simulink model "p2_sync_cosim"  (Simulink 6.4)
settings: Solver=FixedStepDiscrete  SolverMode=SingleTasking  StartTime=0.0  StopTime=0.4  RelTol=1e-3
undefined symbols (not defined in the file or in its folder): pipeline_prec
libraries: modelsimlib x1
settings Model: LastModifiedBy=Administrador

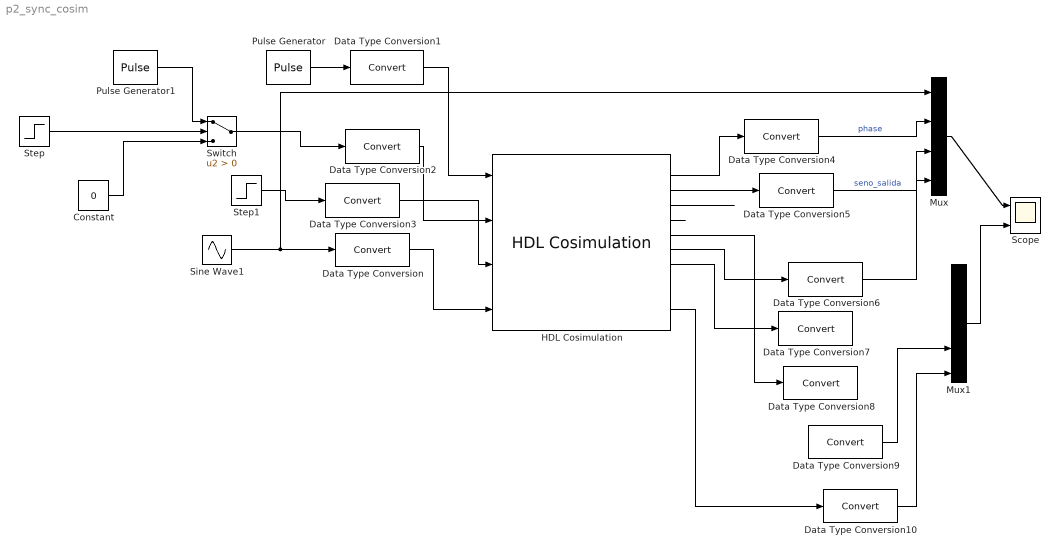
== system p2_sync_cosim ==
  Constant : Constant  Value=0  OutDataType=sfix(16)  ConRadixGroup=Use specified scaling  OutScaling=2^0  SampleTime=-1  FramePeriod=inf
  Data Type Conversion : DataTypeConversion  OutDataTypeMode=Specify via dialog  OutScaling=2^(-pipeline_prec)  RndMeth=Nearest  SaturateOnIntegerOverflow=on
  Data Type Conversion1 : DataTypeConversion  OutDataTypeMode=boolean
  Data Type Conversion{4..10} (7 alike) : DataTypeConversion
  Data Type Conversion2 : DataTypeConversion  OutDataTypeMode=boolean
  Data Type Conversion3 : DataTypeConversion  OutDataTypeMode=boolean
  HDL Cosimulation : modelsimlib/HDL Cosimulation  DialogController=modelsimddg.CoSim  DialogControllerArgs=DataTag0  PortPaths=/p2_sync/clk;/p2_sync/sample;/p2_sync/rst;/p2_sync/in_signal;/p2_sync/phase;/p2_sync/out_signal;/p2_sync/ampl;/p2_sync/done;/p2_sync/freq2phase_out_s;/p2_sync/phase_error_s;/p2_sync/in_cos_mul_out_s;/p2_sync/in_signal_reg_out_s;/p2_sync/sin_speedup_reg_out_s;/p2_sync/cos_speedup_reg_out_s  PortModes=[1 1 1 1 2 2 2 2 2 2 2 2 2 2 ]  PortTimes=[1,1,1,1,1e-5,1e-5,1e-5,1,1e-5,1e-5,1e-5,1e-5,1e-5,1e-5]  PortSigns=[-1 -1 -1 -1 1 1 1 -1 1 1 1 1 1 1 ]  PortFracLengths=[0,0,0,0,pipeline_prec,pipeline_prec,pipeline_prec,0,pipeline_prec,pipeline_prec,pipeline_prec,pipeline_prec,pipeline_prec,pipeline_prec]  CommLocal=on  CommSharedMemory=off  CommPortNumber=4449  CommShowInfo=on  ClockModes=[]  ClockTimes=[]  TclPreSimCommand="echo \"Running Simulink Cosimulation block.\""  TclPostSimCommand="echo \"done\""  TimingMode=s  TimingScaleFactor=1  idxCellArray={'UNUSED_VAR'}
  Mux : Mux
  Mux1 : Mux  Inputs=5
  Pulse Generator : DiscretePulseGenerator  PulseType=Time based  Period=1/(1e6)  PulseWidth=50
  Pulse Generator1 : DiscretePulseGenerator  PulseType=Time based  Period=0.1e-3  PulseWidth=2
  Scope : Scope  NumInputPorts=2
      settings: YMin=-3.5~-1  YMax=3.5~2  MaxDataPoints=500000
  Sine Wave1 : Sin  Frequency=2*pi*50  Phase=1
  Step : Step  Time=4*(1/1e6)
  Step1 : Step  Time=6*(1/1e6)  Before=1  After=0
  Switch : Switch  Criteria=u2 > Threshold  RndMeth=Nearest  ZeroCross=off  SampleTime=1e-7
  wires:
  Data Type Conversion/1 -> HDL Cosimulation/4
  Sine Wave1/1 -> Data Type Conversion/1, Mux/1
  Pulse Generator/1 -> Data Type Conversion1/1
  Data Type Conversion1/1 -> HDL Cosimulation/1
  Switch/1 -> Data Type Conversion2/1
  Data Type Conversion2/1 -> HDL Cosimulation/2
  Step1/1 -> Data Type Conversion3/1
  Data Type Conversion3/1 -> HDL Cosimulation/3
  Constant/1 -> Switch/3
  Step/1 -> Switch/2
  Pulse Generator1/1 -> Switch/1
  Mux/1 -> Scope/1
  HDL Cosimulation/1 -> Data Type Conversion4/1
  Data Type Conversion4/1 -> Mux/2  "phase"
  Data Type Conversion5/1 -> Mux/3  "seno_salida"
  HDL Cosimulation/2 -> Data Type Conversion5/1
  HDL Cosimulation/3 -> ?
  Mux1/1 -> Scope/2
  HDL Cosimulation/4 -> ?
  HDL Cosimulation/6 -> Data Type Conversion6/1
  HDL Cosimulation/7 -> Data Type Conversion7/1
  HDL Cosimulation/5 -> Data Type Conversion8/1
  HDL Cosimulation/10 -> Data Type Conversion10/1
  Data Type Conversion9/1 -> Mux1/4
  Data Type Conversion10/1 -> Mux1/5
  Data Type Conversion6/1 -> Mux/4
